simulink model "statelessSimpleTankTest"  (R2020b)
settings: Solver=VariableStepAuto  StartTime=0.0  StopTime=50  RelTol=1e-3
libraries: nesl_utility x7, fl_lib x1, SimscapeCustomBlocks_lib x1
settings Model: Creator=Edward  LastModifiedBy=Edward

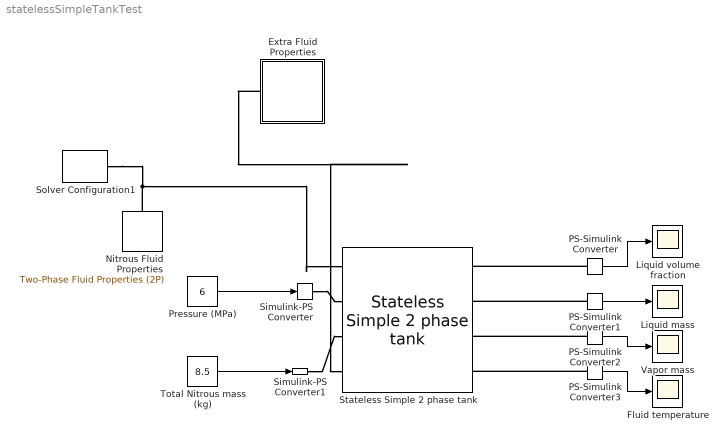
== system statelessSimpleTankTest ==
  Extra Fluid Properties : Subsystem  ReferencedSubsystem=nitrousExtraFluidProps
  Fluid temperature : Scope
  Liquid mass : Scope
  Liquid volume fraction : Scope
  Nitrous Fluid Properties : fl_lib/Two-Phase Fluid/Utilities/Two-Phase Fluid Properties (2P)  u_min=Sim.nitrousFluidTable.u_min kJ/kg  u_max=Sim.nitrousFluidTable.u_max kJ/kg  unorm_liq=Sim.nitrousFluidTable.liquid.unorm  unorm_vap=Sim.nitrousFluidTable.vapor.unorm  p_TLU=Sim.nitrousFluidTable.p MPa  v_liq=Sim.nitrousFluidTable.liquid.v m^3/kg  v_vap=Sim.nitrousFluidTable.vapor.v m^3/kg  s_liq=Sim.nitrousFluidTable.liquid.s kJ/kg/K  s_vap=Sim.nitrousFluidTable.vapor.s kJ/kg/K  T_liq=Sim.nitrousFluidTable.liquid.T K  T_vap=Sim.nitrousFluidTable.vapor.T K  nu_liq=Sim.nitrousFluidTable.liquid.nu mm^2/s  nu_vap=Sim.nitrousFluidTable.vapor.nu mm^2/s  k_liq=Sim.nitrousFluidTable.liquid.k W/(m*K)  k_vap=Sim.nitrousFluidTable.vapor.k W/(m*K)  Pr_liq=Sim.nitrousFluidTable.liquid.Pr  Pr_vap=Sim.nitrousFluidTable.vapor.Pr  u_sat_liq=Sim.nitrousFluidTable.liquid.u_sat kJ/kg  u_sat_vap=Sim.nitrousFluidTable.vapor.u_sat kJ/kg  p_crit=Sim.nitrousFluidTable.p_crit MPa  critical_region=foundation.enum.critical_region.clip  p_crit_fraction=0.12  p_atm=0.101325 MPa  q_rev=0.01 Pa
      settings: SourceProductBaseCode=SS  InternalSimscapePortConfiguration="{\"Bottom\":[],\"Left\":[],\"Right\":[{\"id\":\"A\",\"label\":\"\",\"type\":\"foundation.two_phase_fluid.two_phase_fluid\"}],\"Top\":[]}"
  PS-Simulink Converter{,1..3} (4 alike) : nesl_utility/PS-Simulink Converter  PhysicalDomain=network_engine_domain  SubClassName=ps_output  LeftPortType=input  RightPortType=output  PseudoPeriodic=off  Frequencies=[]  Unit=inherit  AffineConversion=off
  Pressure (MPa) : Constant  Value=6
  Simulink-PS Converter : nesl_utility/Simulink-PS Converter  PhysicalDomain=network_engine_domain  SubClassName=ps_input  LeftPortType=input  RightPortType=output  PseudoPeriodic=off  Frequencies=[]  NoiseDistribution=none  NoiseParameters=[]  Unit=1  AffineConversion=off  FilteringAndDerivatives=provide  SimscapeFilterOrder=1  InputFilterTimeConstant=0.001  UdotUserProvided=0
  Simulink-PS Converter1 : nesl_utility/Simulink-PS Converter  PhysicalDomain=network_engine_domain  SubClassName=ps_input  LeftPortType=input  RightPortType=output  PseudoPeriodic=off  Frequencies=[]  NoiseDistribution=none  NoiseParameters=[]  Unit=1  AffineConversion=off  FilteringAndDerivatives=provide  SimscapeFilterOrder=1  InputFilterTimeConstant=0.001  UdotUserProvided=0
  Solver Configuration1 : nesl_utility/Solver Configuration  PhysicalDomain=network_engine_domain  SubClassName=solver  LeftPortType=input  RightPortType=generic  Tones=[]  Harmonics=[]  SimulateNoise=off  Profile=off  UseLocalSampling=off  EnableSwitchedLinearOptims=on  FrequencyDomain=off  UseCCode=off  RelTol=0.001  AbsTol=1e-06  MinStep=1e-09  ToWorkspace=off  RevertToSquareIcSolve=off  NumHomotopyIterations=100  PhasorMode=off  PhasorModeNumHarmonics=1  DoDC=off  ResidualTolerance=1e-9  UseLocalSolver=off  LocalSolverChoice=NE_BACKWARD_EULER_ADVANCER  LocalSolverSampleTime=0.001  DoFixedCost=off  MaxNonlinIter=3  MaxModeIter=2  ComputeImpulses=off  ImpulseIterations=2  LinearAlgebra=auto  EquationFormulation=NE_TIME_EF  DelaysMemoryBudget=1024  AutomaticFiltering=on  FilteringTimeConstant=0.001  PartitionStorageMethod=AS_NEEDED  PartitionMemoryBudget=1024  PartitionMethod=ROBUST
  Stateless Simple 2 phase tank : SimscapeCustomBlocks_lib/Stateless Simple 2 phase tank  areaL=0.01 m^2  tank_volume=Sim.runTank.volume m^3
      settings: InternalSimscapePortConfiguration="{\"Bottom\":[],\"Left\":[{\"id\":\"N\",\"label\":\"2P_Props\",\"type\":\"foundation.two_phase_fluid.two_phase_fluid\"},{\"id\":\"p_tank\",\"label\":\"P\",\"type\":\"input\"},{\"id\":\"totalFluidMass\",\"label\":\"M\",\"type\":\"input\"}],\"Right\":[{\"id\":\"L\",\"label\":\"L\",\"type\":\"output\"},{\"id\":\"ML\",\"label\":\"ML\",\"type\":\"output\"},{\"id\":\"MV\",\"label\":\"MV\",\"type\":\"output\"},{\"id\":\"T\",\"label\":\"T\",\"type\":\"output\"}],\"Top\":[{\"id\":\"Props\",\"label\":\"Props\",\"type\":\"SimscapeCustomBlocks.customFluidDomain.extra_two_phase_fluid_props\"}]}"
  Total Nitrous mass (kg) : Constant  Value=8.5
  Vapor mass : Scope
  wires:
  Pressure (MPa)/1 -> Simulink-PS Converter/1
  Total Nitrous mass (kg)/1 -> Simulink-PS Converter1/1
  PS-Simulink Converter/1 -> Liquid volume fraction/1
  PS-Simulink Converter1/1 -> Liquid mass/1
  PS-Simulink Converter2/1 -> Vapor mass/1
  PS-Simulink Converter3/1 -> Fluid temperature/1
  connections:
  Nitrous Fluid Properties/RConn1 -- Solver Configuration1/RConn1 -- Stateless Simple 2 phase tank/LConn1
  Extra Fluid Properties/RConn1 -- Stateless Simple 2 phase tank/LConn4
  Simulink-PS Converter/RConn1 -- Stateless Simple 2 phase tank/LConn2
  Simulink-PS Converter1/RConn1 -- Stateless Simple 2 phase tank/LConn3
  PS-Simulink Converter/LConn1 -- Stateless Simple 2 phase tank/RConn1
  PS-Simulink Converter1/LConn1 -- Stateless Simple 2 phase tank/RConn2
  PS-Simulink Converter2/LConn1 -- Stateless Simple 2 phase tank/RConn3
  PS-Simulink Converter3/LConn1 -- Stateless Simple 2 phase tank/RConn4
